simulink model "chariot"  (R2025a)
settings: Solver=VariableStepAuto  StartTime=0.0  StopTime=30.0  RelTol=1e-3
values from neighbouring files (symbols this model uses):
  a = 250e3    (= 250000)    [bateau_data.m]    (also in chariot_data.m; porte_avion.m)
  A_ch = [0 1 ... (first row only)    [chariot_data.m]
  B_ch = [0 ... (first row only)    [chariot_data.m]
  C_ch = [1 0]    [chariot_data.m]
  D_ch = 0    [chariot_data.m]
  g = 9.81    [bateau_data.m]    (also in chariot_data.m; porte_avion.m)
settings Model: Creator=vikfo  LastModifiedBy=vikfo

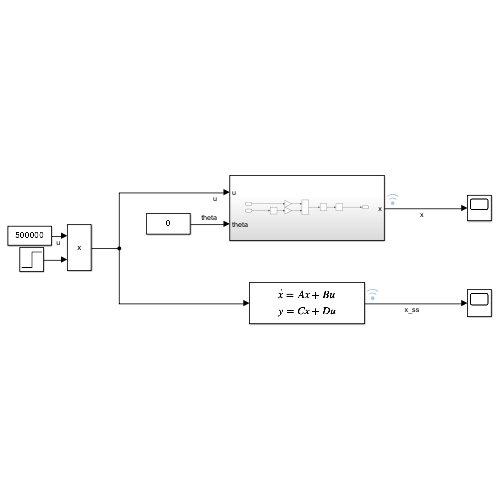
[thumbnail: Simulink's stored preview of the top-level diagram]
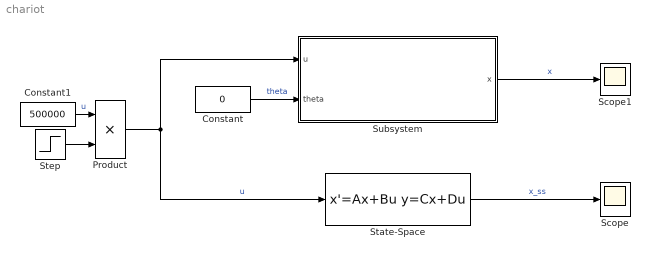
== system chariot ==
  Constant : Constant  Value=0
  Constant1 : Constant  Value=500000
  Product : Product
  Scope : Scope
      settings: ActiveDisplayYMinimum=-1  ActiveDisplayYMaximum=1
  Scope1 : Scope
      settings: ActiveDisplayYMinimum=-1  ActiveDisplayYMaximum=1
  State-Space : StateSpace  A=A_ch  B=B_ch  C=C_ch  D=D_ch  InitialCondition=0
  Step : Step  SampleTime=0
  Subsystem : Subsystem
  wires:
  State-Space/1 -> Scope/1  "x_ss"
  Product/1 -> State-Space/1, Subsystem/1(u)  "u"
  Constant/1 -> Subsystem/2(theta)  "theta"
  Subsystem/1(x) -> Scope1/1  "x"
  Constant1/1 -> Product/1  "u"
  Step/1 -> Product/2

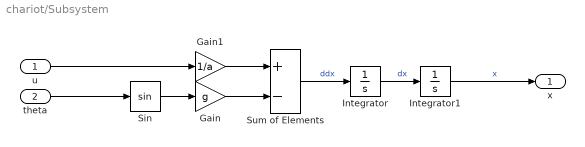
== system chariot/Subsystem ==
  u : Inport
  theta : Inport  Port=2
  Gain : Gain  Gain=g
  Gain1 : Gain  Gain=1/a
  Integrator : Integrator
  Integrator1 : Integrator
  Sin : Trigonometry
  Sum of Elements : Sum  Inputs=+-
  x : Outport
  wires:
  Integrator/1 -> Integrator1/1  "dx"
  Integrator1/1 -> x/1  "x"
  Sin/1 -> Gain/1
  Sum of Elements/1 -> Integrator/1  "ddx"
  Gain/1 -> Sum of Elements/2
  u/1 -> Gain1/1
  Gain1/1 -> Sum of Elements/1
  theta/1 -> Sin/1
